simulink model "Model_Room"  (R2020a)
settings: Solver=VariableStepAuto  StartTime=0.0  StopTime=365*24  RelTol=1e-3
settings Model: Creator=HP  LastModifiedBy=carlo
settings DebuggingCC: ArithmeticOperatorsInVariantConditions=warning
settings SFSimCC: CustomCodeUndefinedFunction=UseInterfaceOnly

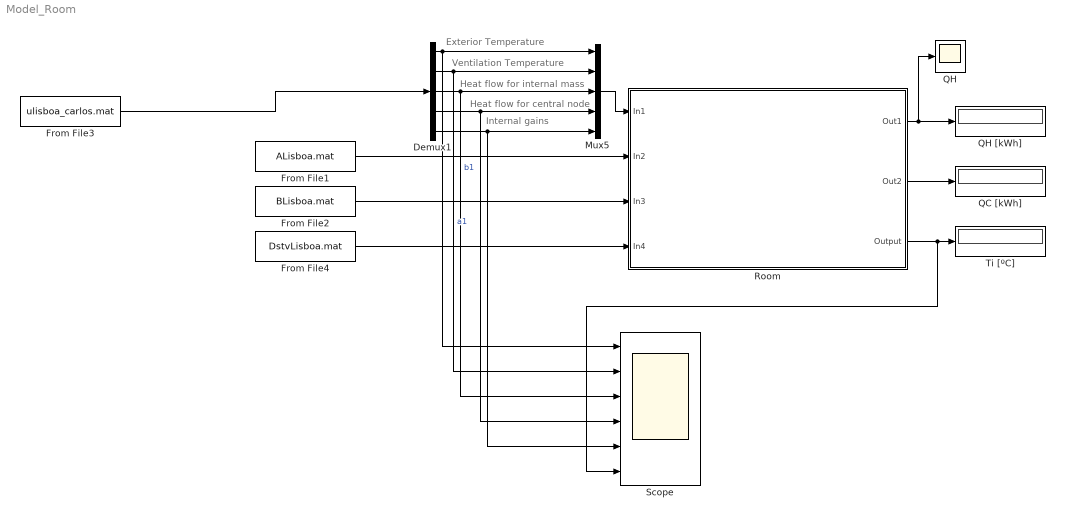
== system Model_Room ==
  note: Internal gains
  note: Exterior Temperature
  note: Ventilation Temperature
  note: Heat flow for internal mass
  note: Heat flow for central node
  Demux1 : Demux  Outputs=[1 1 1 1 1]
  From File1 : FromFile  FileName=ALisboa.mat  SampleTime=1
  From File2 : FromFile  FileName=BLisboa.mat  SampleTime=1
  From File3 : FromFile  FileName=ulisboa_carlos.mat  SampleTime=1
  From File4 : FromFile  FileName=DstvLisboa.mat  SampleTime=1
  Mux5 : Mux  Inputs=5
  QC [kWh] : Display
      settings: Format=bank  SampleTime=1
  QH : Scope
  QH [kWh] : Display
      settings: Format=bank  SampleTime=1
  Room : Subsystem
      mask Display: image('roomoffice.jpg'); % Use "Edit Image" on toolstrip to change.
  Scope : Scope  NumInputPorts=6
  Ti [ºC] : Display
      settings: Format=bank  SampleTime=1
  wires:
  Mux5/1 -> Room/1(In1)
  Room/3(Output) -> Scope/6, Ti [ºC]/1
  Demux1/3 -> Scope/3, Mux5/3  "b1"
  From File4/1 -> Room/4(In4)
  Demux1/2 -> Scope/2, Mux5/2  "a1"
  Room/1(Out1) -> QH/1, QH [kWh]/1
  From File1/1 -> Room/2(In2)
  From File2/1 -> Room/3(In3)
  Room/2(Out2) -> QC [kWh]/1
  Demux1/1 -> Scope/1, Mux5/1
  From File3/1 -> Demux1/1
  Demux1/5 -> Scope/5, Mux5/5
  Demux1/4 -> Scope/4, Mux5/4

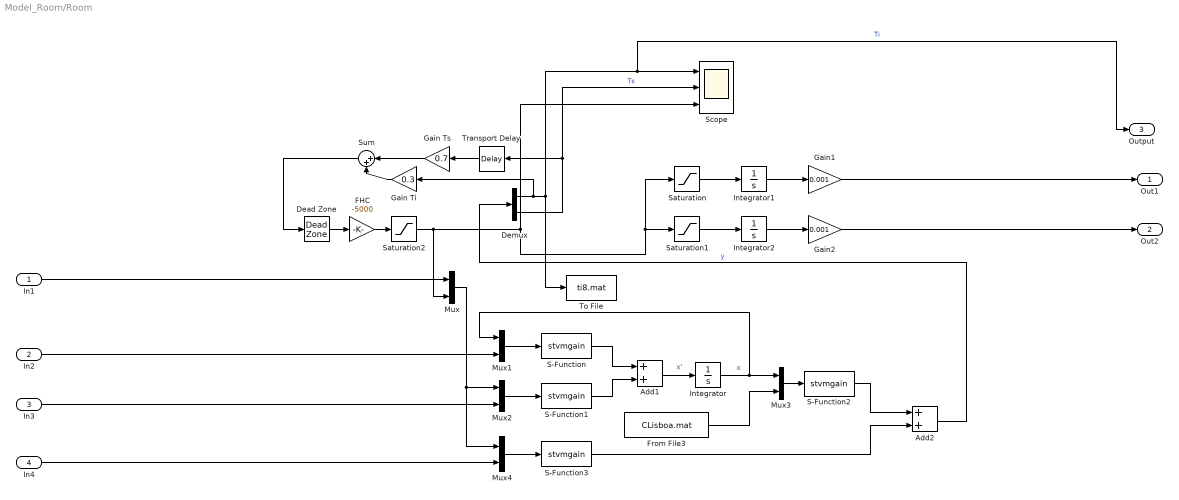
== system Model_Room/Room ==
  note: x'
  note: x
  In1 : Inport
  In2 : Inport  Port=2
  In3 : Inport  Port=3
  In4 : Inport  Port=4
  Add1 : Sum
  Add2 : Sum
  Dead Zone : DeadZone  LowerValue=20  UpperValue=26  ZeroCross=off  SaturateOnIntegerOverflow=on
  Demux : Demux  Outputs=2
  FHC : Gain  Gain=-5000
  From File3 : FromFile  FileName=CLisboa.mat  SampleTime=1
  Gain Ti : Gain  Gain=0.3
  Gain Ts : Gain  Gain=0.7
  Gain1 : Gain  Gain=0.001  SampleTime=1
  Gain2 : Gain  Gain=0.001  SampleTime=1
  Integrator : Integrator  InitialCondition=18
  Integrator1 : Integrator
  Integrator2 : Integrator
  Mux : Mux  Inputs=2
  Mux1 : Mux  Inputs=[1 1]
  Mux2 : Mux  Inputs=[6 6]
  Mux3 : Mux  Inputs=[1 2]
  Mux4 : Mux  Inputs=[6 12]
  S-Function : S-Function  FunctionName=stvmgain  Parameters=1, -1  SFunctionDeploymentMode=off  EnableBusSupport=off
  S-Function1 : S-Function  FunctionName=stvmgain  Parameters=[1 1 1 1 1 1], -1  SFunctionDeploymentMode=off  EnableBusSupport=off
  S-Function2 : S-Function  FunctionName=stvmgain  Parameters=[1 ;1] -1  SFunctionDeploymentMode=off  EnableBusSupport=off
  S-Function3 : S-Function  FunctionName=stvmgain  Parameters=[1 1 1 1 1 1; 1 1 1 1 1 1], -1  SFunctionDeploymentMode=off  EnableBusSupport=off
  Saturation : Saturate  UpperLimit=20000  LowerLimit=0  SampleTime=1
  Saturation1 : Saturate  UpperLimit=0  LowerLimit=-20000  SampleTime=1
  Saturation2 : Saturate  UpperLimit=10000  LowerLimit=-10000
  Scope : Scope  NumInputPorts=3
  Sum : Sum  Inputs=|++
  To File : ToFile  Filename=ti8.mat  SampleTime=1
  Transport Delay : TransportDelay
  Out1 : Outport  VectorParamsAs1DForOutWhenUnconnected=off
  Out2 : Outport  Port=2  VectorParamsAs1DForOutWhenUnconnected=off
  Output : Outport  Port=3  VectorParamsAs1DForOutWhenUnconnected=off
  wires:
  Sum/1 -> Dead Zone/1
  Mux3/1 -> S-Function2/1
  Demux/1 -> Gain Ti/1, Output/1, Scope/1, To File/1  "Ti"
  Mux2/1 -> S-Function1/1
  Saturation2/1 -> Mux/2, Scope/3, Saturation1/1, Saturation/1
  Mux/1 -> Mux2/1, Mux4/1
  Saturation/1 -> Integrator1/1
  Gain1/1 -> Out1/1
  S-Function/1 -> Add1/1
  Mux4/1 -> S-Function3/1
  Integrator/1 -> Mux3/1, Mux1/1
  FHC/1 -> Saturation2/1
  Saturation1/1 -> Integrator2/1
  Gain Ts/1 -> Sum/1
  Mux1/1 -> S-Function/1
  S-Function3/1 -> Add2/2
  Transport Delay/1 -> Gain Ts/1
  Dead Zone/1 -> FHC/1
  Gain Ti/1 -> Sum/2
  S-Function1/1 -> Add1/2
  Integrator2/1 -> Gain2/1
  Demux/2 -> Scope/2, Transport Delay/1  "Ts"
  In3/1 -> Mux2/2
  Add1/1 -> Integrator/1
  Gain2/1 -> Out2/1
  From File3/1 -> Mux3/2
  In2/1 -> Mux1/2
  S-Function2/1 -> Add2/1
  Integrator1/1 -> Gain1/1
  Add2/1 -> Demux/1  "y"
  In4/1 -> Mux4/2
  In1/1 -> Mux/1
